simulink model "L15SimPend"  (R2022b)
settings: Solver=FixedStepAuto  StartTime=0.0  StopTime=10.0  FixedStep=0.01  RelTol=1e-3
InitFcn:
  | L15ParametersPend;
values from neighbouring files (symbols this model uses):
  A = [0 1 ; g/l -r/(m*l^2)]    [L15ParametersPend.m]
  B = [0 ; 1/(m*l^2)]    [L15ParametersPend.m]
  K = lqr(A,B,Q,R)    [L15ParametersPend.m]
  x0 = [theta0 ; thetadot0]    [L15ParametersPend.m]
settings Model: Creator=vcichella  LastModifiedBy=vcichella
settings SolverCC: AlgebraicLoopSolver=TrustRegion
settings DebuggingCC: UnconnectedInputMsg=warning  UnconnectedOutputMsg=warning  UnconnectedLineMsg=warning  SFMachineParentedDataDiag=warning
settings ModelReferenceCC: EnableRefExpFcnMdlSchedulingChecks=on
settings RTWCC: DLArmComputeVersion=19.05

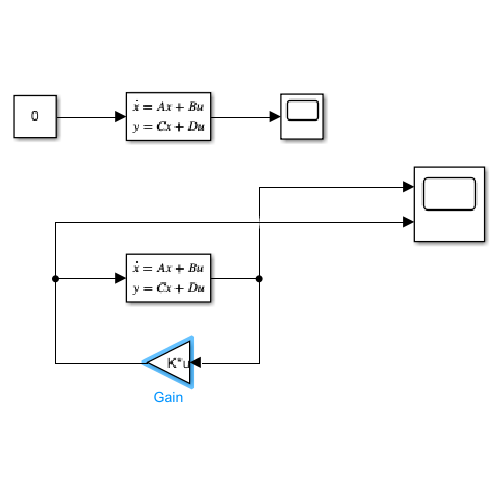
[thumbnail: Simulink's stored preview of the top-level diagram]
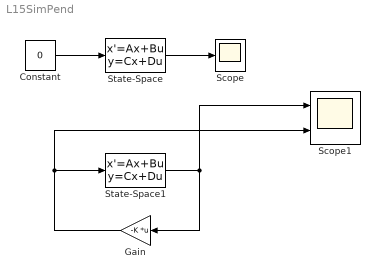
== system L15SimPend ==
  Constant : Constant  Value=0
  Gain : Gain  Gain=-K  Multiplication=Matrix(K*u)
  Scope : Scope
  Scope1 : Scope  NumInputPorts=2
  State-Space : StateSpace  A=A  B=B  C=eye(2)  D=zeros(2,1)  InitialCondition=x0
  State-Space1 : StateSpace  A=A  B=B  C=eye(2)  D=zeros(2,1)  InitialCondition=x0
  wires:
  Constant/1 -> State-Space/1
  State-Space/1 -> Scope/1
  State-Space1/1 -> Gain/1, Scope1/1
  Gain/1 -> Scope1/2, State-Space1/1
